simulink model "joint_test_dis_massless"  (R2015a)
settings: Solver=ode45  SolverMode=SingleTasking  StartTime=0.0  StopTime=10.0  RelTol=1e-3
libraries: mblibv1 x13
Description:
  | Copyright 2014 The MathWorks, Inc.
settings Model: Creator=smiller  LastModifiedBy=smiller
settings DataIOCC: SignalLoggingSaveFormat=ModelDataLogs
settings OptimizationCC: BlockReduction=off  BooleanDataType=off
settings DebuggingCC: SaveWithParameterizedLinksMsg=none  UnderspecifiedInitializationDetection=Classic  MergeDetectMultiDrivingBlocksExec=none  SignalResolutionControl=TryResolveAllWithWarning  MultiTaskDSMMsg=warning  MultiTaskCondExecSysMsg=none  StateNameClashWarn=warning  StrictBusMsg=None
settings HardwareCC: TargetUnknown=on

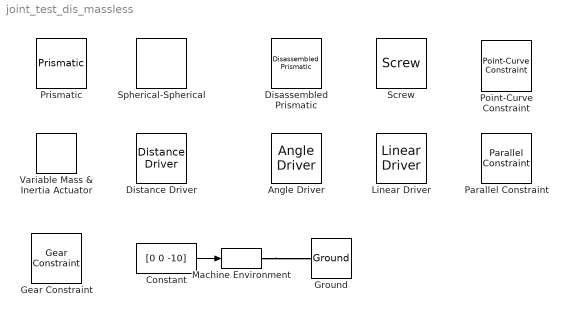
== system joint_test_dis_massless ==
  Angle Driver : mblibv1/Constraints &  Drivers/Angle Driver  LConnTagsString=__newl0  RConnTagsString=__newr0  UpdateFromCAD=off  DialogClass=AngleDriverConstraint  NumSAPorts=0  LeftCsys=WORLD  RightCsys=WORLD  LeftAxis=[1 0 0]  RightAxis=[1 0 0]
  Constant : Constant  Value=[0 0 -10]
  Disassembled Prismatic : mblibv1/Joints/Disassembled Joints/Disassembled Prismatic  LConnTagsString=__newl0  RConnTagsString=__newr0  UpdateFromCAD=off  DialogClass=JointBlock  Primitives=prismatic  PrimitiveProps=Base$WORLD$[1 0 0]$prismatic#Follower$WORLD$[0 1 0]$prismatic  BaseAxis=[1 0 0]  FollowerAxis=[0 1 0]
  Distance Driver : mblibv1/Constraints &  Drivers/Distance Driver  LConnTagsString=__newl0  RConnTagsString=__newr0  UpdateFromCAD=off  DialogClass=DistanceDriverConstraint  NumSAPorts=0
  Gear Constraint : mblibv1/Constraints &  Drivers/Gear Constraint  LConnTagsString=__newl0  RConnTagsString=__newr0  UpdateFromCAD=off  DialogClass=GearConstraint  NumSAPorts=0  BaseRadius=1  BaseRadiusUnits=m  FollowerRadius=1  FollowerRadiusUnits=m
  Ground : mblibv1/Bodies/Ground  UpdateFromCAD=off  LeftPortType=env  RightPortType=workingframe  PhysicalDomain=Mechanical  DialogClass=GroundBlock  CoordPosition=[0 0 0]  CoordPositionUnits=m  StateVectorMgrId=-1  MachineId=[0 0]  ShowEnvPort=on  ParameterChecksum=[0 0 0 0]  TopologyChecksum=[0 0 0 0]
  Linear Driver : mblibv1/Constraints &  Drivers/Linear Driver  LConnTagsString=__newl0  RConnTagsString=__newr0  UpdateFromCAD=off  DialogClass=LinearDriverConstraint  NumSAPorts=0  GlobalCoordinate=X
  Machine Environment : mblibv1/Bodies/Machine Environment  PortType=env  PhysicalDomain=Mechanical  DialogTemplateClass=MECH.MachineEnvironment  SyncWhenCopied=off  Gravity=[0 -9.81 0]  GravityUnits=m/s^2  GravityAsSignal=on  Dimensionality=Auto-detect  AnalysisType=Forward dynamics  LinearAssemblyTolerance=1e-3  LinearAssemblyToleranceUnits=m  AngularAssemblyTolerance=1e-3  AngularAssemblyToleranceUnits=rad  ConstraintSolverType=Stabilizing  ConstraintRelTolerance=1e-4  ConstraintAbsTolerance=1e-4  UseRobustSingularityHandling=off  RedundancyAnalysisToleranceType=Automatically select tolerance  RedundancyAnalysisTolerance=1e-14  StatePerturbationType=Fixed  PerturbationSize=1e-5  VisualizeMachine=on  BodyVisualizationType=Use model default body geometries  BodyColorSelMode=Use model default  DefaultBodyColor=[1 0 0]
  Parallel Constraint : mblibv1/Constraints &  Drivers/Parallel Constraint  LConnTagsString=__newl0  RConnTagsString=__newr0  UpdateFromCAD=off  DialogClass=ParallelConstraint  NumSAPorts=0  Csys=WORLD  Axis=[1 0 0]
  Point-Curve Constraint : mblibv1/Constraints &  Drivers/Point-Curve Constraint  LConnTagsString=__newl0|SA1  RConnTagsString=__newr0  UpdateFromCAD=off  DialogClass=PointCurveConstraint  Units=m  Xbreaks="[1     0.77547    0.058989    -0.52528    -0.55899    -0.17022     0.65485]"  Ybreaks="[0     0.42955     0.56832     0.29503    -0.12733    -0.36512    -0.39199]"  Zbreaks="[-0.0031056     0.36957     0.56832     0.29503    -0.12733    -0.46273    -0.40062]*0"  EndConditions=periodic  CanExtrapolate=off  NumSAPorts=1
  Prismatic : mblibv1/Joints/Prismatic  LConnTagsString=__newl0  RConnTagsString=__newr0  UpdateFromCAD=off  NumSAPorts=0  CutJoint=off  MarkAsCut=off  Primitives=prismatic  PrimitiveProps=P1$World$[1 0 0]$prismatic  DialogClass=JointBlock  P1Axis=[1 0 0]
  Screw : mblibv1/Joints/Screw  LConnTagsString=__newl0  RConnTagsString=__newr0  UpdateFromCAD=off  NumSAPorts=0  CutJoint=off  MarkAsCut=off  Primitives=prismatic  PrimitiveProps=R1$WORLD$[1 0 0]$revolute  DialogClass=ScrewJointBlock  Pitch=1  Units=mm  R1Axis=[1 0 0]
  Spherical-Spherical : mblibv1/Joints/Massless Connectors/Spherical-Spherical  LConnTagsString=__newl0  RConnTagsString=__newr0  UpdateFromCAD=off  NumSAPorts=0  CutJoint=off  MarkAsCut=off  Primitives=prismatic  PrimitiveProps=S1$WORLD$[0 0 0]$spherical#S2$WORLD$[0 0 0]$spherical  DialogClass=JointBlock  S1Axis=[0 0 0]  S2Axis=[0 0 0]
  Variable Mass & Inertia Actuator : mblibv1/Sensors &  Actuators/Variable Mass & Inertia Actuator  UpdateFromCAD=off  PhysicalDomain=Mechanical  PortType=blob  ActuationStyle=MassInertia  AngleUnits=deg  ArcVelocityUnits=deg/s  ArcAccelerationUnits=deg/s^2  CoordPositionUnits=m  VelocityUnits=m/s  AccelerationUnits=m/s^2  ForceUnits=N  TorqueUnits=N-m  ActiveIO=off  Width=1  DialogClass=VariableMassInertiaActuatorBlock  Mass=on  Inertia=off  ReferenceFrame=Local (body CS)  MassUnits=kg  InertiaUnits=kg*m^2
  wires:
  Constant/1 -> Machine Environment/1
  connections:
  Machine Environment/RConn1 -- Ground/LConn1
